simulink model "node23_case_10kV_withLoad_v2"  (R2022b)
settings: Solver=VariableStepAuto  StartTime=0.0  StopTime=10  FixedStep=1e-6  RelTol=1e-5
InitFcn:
  | sw=5;
  | Lf=1.75e-3+3.5e-3;
  | %Lf=3.5e-3;
  | %Cf=2e-4;
  | f=10;
  | Cf=15e-6;
  | % L=1.75e-3/2;
  | % X=100*pi*L;
  | % R=2*X;
  | R=0.25;X=R/0.66;
  | L=X/100/pi;
  | Z=sqrt(R^2+X^2);
  | f = 30;
  | kp1=10;
  | ki1=100;
  | kp4=20;
  | ki4=100;
  | kp16=20;
  | ki16=100;
  | % 负载参数
  | R1L=0;
  | X1L=0;
  | R2L=652.4467;
  | X2L=276.0351;
  | R3L=804.5741;
  | X3L=256.7790;
  | R4L=760.9867;
  | X4L=234.6376;
  | R5L=818.7384;
  | X5L=266.9799;
  | R6L=671.1329;
  | X6L=170.1801;
  | R7L=883.7621;
  | X7L=178.8663;
  | R8L=388.3725;
  | X8L=158.3040;
  | R9L=817.4819;
  | X9L=268.6933;
  | R10L=849.4733;
  | X10L=254.8420;
  | R11L=407.8415;
  | X11L=165.8504;
  | R12L=NaN;  % Bus 12 无 R、X 数据，用 NaN 标记
  | X12L=NaN;
  | R13L=751.2339;
  | X13L=329.8428;
  | R14L=294.0393;
  | X14L=141.6929;
  | R15L=761.9027;
  | X15L=284.3908;
  | R16L=740.4040;
  | X16L=318.2438;
  | R17L=674.5784;
  | X17L=316.4689;
  | R18L=776.7449;
  | X18L=316.6080;
  | R19L=766.0423;
  | X19L=335.7994;
  | R20L=746.0545;
  | X20L=344.3329;
  | ... (+266 lines)
libraries: spsSeriesRLCBranchLib x210, slpidlib x45, spsControlledVoltageSourceLib x30, spsThreePhaseVIMeasurementLib x24, spsPower3phInstantaneousLib x13, spsAlphaBetaZerotoabcLib x9, spsCurrentMeasurementLib x6, spsGroundLib x2, spspowerguiLib x1
(part 2 of 8)

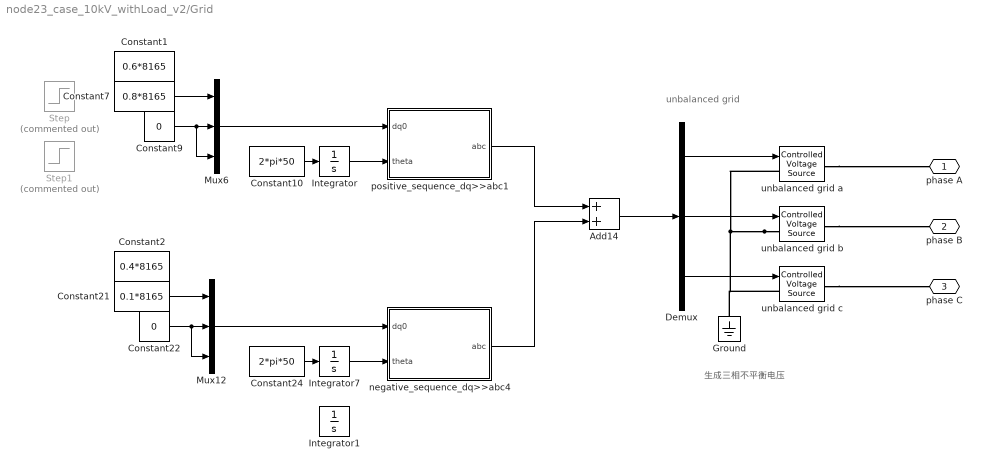
== system node23_case_10kV_withLoad_v2/Grid ==
  note: unbalanced grid
  note: 生成三相不平衡电压
  Add14 : Sum
  Constant1 : Constant  Value=0.6*8165
  Constant10 : Constant  Value=2*pi*50
  Constant2 : Constant  Value=0.4*8165
  Constant21 : Constant  Value=0.1*8165
  Constant22 : Constant  Value=0
  Constant24 : Constant  Value=2*pi*50
  Constant7 : Constant  Value=0.8*8165
  Constant9 : Constant  Value=0
  Demux : Demux  Outputs=3
  Ground : spsGroundLib/Ground  LConnTagsString=a
  Integrator : Integrator
  Integrator1 : Integrator  InitialCondition=-pi/6
  Integrator7 : Integrator  InitialCondition=-pi/2
  Mux12 : Mux  Inputs=3
  Mux6 : Mux  Inputs=3
  Step : Step  Commented=on  Time=0.25  Before=311  After=280  SampleTime=0
  Step1 : Step  Commented=on  Time=0.25  After=100  SampleTime=0
  negative_sequence_dq>>abc4 : Subsystem
  positive_sequence_dq>>abc1 : Subsystem
  unbalanced grid a : spsControlledVoltageSourceLib/Controlled Voltage Source  Initialize=on  Source_Type=AC  Amplitude=0  Phase=0  Frequency=0  Measurements=None
  "unbalanced grid b " : spsControlledVoltageSourceLib/Controlled Voltage Source  Initialize=on  Source_Type=AC  Amplitude=0  Phase=0  Frequency=0  Measurements=None
  unbalanced grid c : spsControlledVoltageSourceLib/Controlled Voltage Source  Initialize=on  Source_Type=AC  Amplitude=0  Phase=0  Frequency=0  Measurements=None
  phase A : PMIOPort  Side=Right
  phase B : PMIOPort  Port=2  Side=Right
  phase C : PMIOPort  Port=3  Side=Right
  wires:
  negative_sequence_dq>>abc4/1(abc) -> Add14/2
  Mux12/1 -> negative_sequence_dq>>abc4/1(dq0)
  Integrator/1 -> positive_sequence_dq>>abc1/2(theta)
  Demux/2 -> "unbalanced grid b "/1
  Constant24/1 -> Integrator7/1
  positive_sequence_dq>>abc1/1(abc) -> Add14/1
  Constant9/1 -> Mux6/3, Mux6/2
  Mux6/1 -> positive_sequence_dq>>abc1/1(dq0)
  Constant10/1 -> Integrator/1
  Demux/3 -> unbalanced grid c/1
  Demux/1 -> unbalanced grid a/1
  Integrator7/1 -> negative_sequence_dq>>abc4/2(theta)
  Add14/1 -> Demux/1
  Constant22/1 -> Mux12/3, Mux12/2
  Constant7/1 -> Mux6/1
  Constant21/1 -> Mux12/1
  connections:
  unbalanced grid c/RConn1 -- phase C/RConn1
  "unbalanced grid b "/LConn1 -- Ground/LConn1 -- unbalanced grid c/LConn1 -- unbalanced grid a/LConn1
  "unbalanced grid b "/RConn1 -- phase B/RConn1
  unbalanced grid a/RConn1 -- phase A/RConn1

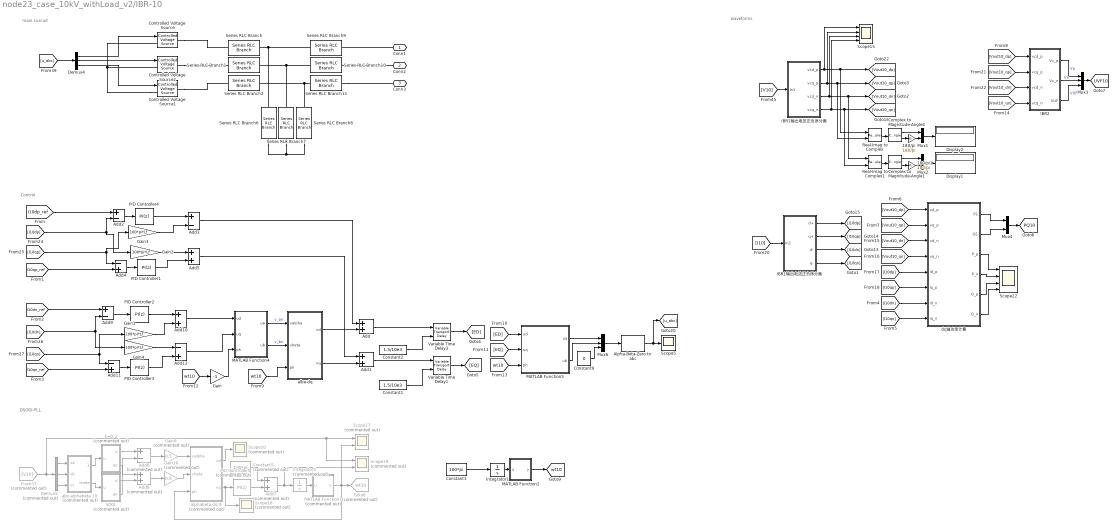
== system node23_case_10kV_withLoad_v2/IBR-10 ==
  note: DSOGI-PLL
  note: main curcuit
  note: Control
  note: waveforms
  180/pi : Gain  Gain=180/pi
  180/pi1 : Gain  Gain=180/pi
  Add{,1,5,10} (4 alike) : Sum
  Add11 : Sum  Inputs=-+
  Add12 : Sum  Inputs=-+
  Add2 : Sum  Inputs=+-
  Add3 : Sum  Inputs=+-
  Add4 : Sum  Inputs=-+
  Add6 : Sum  Commented=on  Inputs=+-
  Add7 : Sum  Commented=on
  Add8 : Sum  Commented=on
  Add9 : Sum  Inputs=+-
  Alpha-Beta-Zero to abc : spsAlphaBetaZerotoabcLib/Alpha-Beta-Zero to abc
      settings: LibrarySourceBlock=|
      | sps_lib/Control/Alpha-Beta-Zero
      | to abc
  Complex to Magnitude-Angle1 : ComplexToMagnitudeAngle
  Complex to Magnitude-Angle4 : ComplexToMagnitudeAngle
  Constant1 : Constant  Value=1.5/10e3
  Constant2 : Constant  Value=1.5/10e3
  Constant3 : Constant  Value=100*pi
  Constant5 : Constant  Commented=on  Value=100*pi
  Constant9 : Constant  Value=0
  Controlled Voltage Source : spsControlledVoltageSourceLib/Controlled Voltage Source  Initialize=on  Source_Type=AC  Amplitude=0  Phase=0  Frequency=0  Measurements=None
  Controlled Voltage Source1 : spsControlledVoltageSourceLib/Controlled Voltage Source  Initialize=on  Source_Type=AC  Amplitude=0  Phase=0  Frequency=0  Measurements=None
  Controlled Voltage Source2 : spsControlledVoltageSourceLib/Controlled Voltage Source  Initialize=on  Source_Type=AC  Amplitude=0  Phase=0  Frequency=0  Measurements=None
  Demux4 : Demux  Outputs=3
  Demux5 : Demux  Commented=on  Outputs=3
  Display1 : Display
  Display2 : Display
  From37 : From  Commented=on  GotoTag=V10  TagVisibility=global
  Gain : Gain  Gain=-1
  Gain{1..4} (4 alike) : Gain  Gain=100*pi*Lf
  Gain10 : Gain  Commented=on  Gain=0.5
  Gain9 : Gain  Commented=on  Gain=0.5
  Goto8 : Goto  Commented=on  GotoTag=wt10  TagVisibility=global
  IBR1输出电压正负序分离 : Subsystem
  IBR1输出电流正负序分离 : Subsystem
  IBR2 : MATLAB Function  TreatAsAtomicUnit=on
  Integrator1 : Integrator
  Integrator5 : Integrator  Commented=on
  MATLAB Function1 : MATLAB Function  Commented=on  TreatAsAtomicUnit=on
  MATLAB Function2 : MATLAB Function  TreatAsAtomicUnit=on
  MATLAB Function4 : MATLAB Function  TreatAsAtomicUnit=on
  MATLAB Function5 : MATLAB Function  TreatAsAtomicUnit=on
  Mux1 : Mux  Inputs=2
  Mux2 : Mux  Inputs=2
  Mux3 : Mux  Inputs=3
  Mux4 : Mux  Inputs=2
  Mux6 : Mux  Inputs=3
  PID Controller{1..4} (4 alike) : slpidlib/PID Controller  Controller=PI  Form=Parallel  TimeDomain=Discrete-time  UseExternalTs=off  SampleTime=-1  IntegratorMethod=Forward Euler  FilterMethod=Forward Euler  ControllerParametersSource=internal  P=kp1  I=ki1  UseKiTs=off  D=0  N=100  UseFilter=on  TunerSelectOption=Transfer Function Based (PID Tuner App)  InitialConditionSource=internal  InitialConditionForIntegrator=0  InitialConditionForFilter=0  DifferentiatorICPrevScaledInput=0  ExternalReset=none  TrackingMode=off  Kt=1  LimitOutput=off  SatLimitsSource=internal  UpperSaturationLimit=5  LowerSaturationLimit=-5  LinearizeAsGain=on  AntiWindupMode=none  Kb=1  LimitIntegrator=off  UpperIntegratorSaturationLimit=inf  LowerIntegratorSaturationLimit=-inf  POutMin=[]  POutMax=[]  IOutMin=[]  IOutMax=[]  DOutMin=[]  DOutMax=[]  NOutMin=[]  NOutMax=[]  SumOutMin=[]  SumOutMax=[]  SaturationOutMin=[]  SaturationOutMax=[]  PParamMin=[]  PParamMax=[]  IParamMin=[]  IParamMax=[]  DParamMin=[]  DParamMax=[]  NParamMin=[]  NParamMax=[]  KbParamMin=[]  KbParamMax=[]  KtParamMin=[]  KtParamMax=[]  KbOutMin=[]  KbOutMax=[]  KtOutMin=[]  KtOutMax=[]  IntegratorOutMin=[]  IntegratorOutMax=[]  FilterOutMin=[]  FilterOutMax=[]  SumI1OutMin=[]  SumI1OutMax=[]  SumI2OutMin=[]  SumI2OutMax=[]  SumI3OutMin=[]  SumI3OutMax=[]  SumI4OutMin=[]  SumI4OutMax=[]  SumDOutMin=[]  SumDOutMax=[]  DifferentiatorOutMin=[]  DifferentiatorOutMax=[]  FilterDiffOutCoefMin=[]  FilterDiffOutCoefMax=[]  ReciprocalOutMin=[]  ReciprocalOutMax=[]  SumDenOutMin=[]  SumDenOutMax=[]  SumNumOutMin=[]  SumNumOutMax=[]  DivideOutMin=[]  DivideOutMax=[]  UdiffTsProdOutMin=[]  UdiffTsProdOutMax=[]  NTsProdOutMin=[]  NTsProdOutMax=[]  UintegralTsProdOutMin=[]  UintegralTsProdOutMax=[]  UngainTsProdOutMin=[]  UngainTsProdOutMax=[]  ClampingZeroOutDataTypeStr=Inherit: Inherit via back propagation  ClampingZeroOutMin=[]  ClampingZeroOutMax=[]  FilterDenConstantOutDataTypeStr=Inherit: Inherit via back propagation  FilterDenConstantOutMin=[]  FilterDenConstantOutMax=[]  PCopyOutDataTypeStr=Inherit: Inherit via back propagation  PCopyOutMin=[]  PCopyOutMax=[]  NCopyOutDataTypeStr=Inherit: Inherit via back propagation  NCopyOutMin=[]  NCopyOutMax=[]  IntegratorContinuousStateAttributes=''  IntegratorStateMustResolveToSignalObject=off  IntegratorRTWStateStorageClass=Auto  FilterContinuousStateAttributes=''  FilterStateMustResolveToSignalObject=off  FilterRTWStateStorageClass=Auto  ParallelPVariant=InternalParameters  IdealPVariant=Disabled  IVariant=InternalParameters  DVariant=Disabled  IntegratorVariant=Discrete  SatVariant=Disabled  AWVariant=Passthrough  PCopyVariant=Disabled  TRVariant=Disabled  FdbkBlocksVariant=Forward  IdealPFdbkVariant=Disabled  SatFdbkVariant=Disabled  DerivativeFilterVariant=Disabled  NVariant=Disabled  NCopyVariant=Disabled_SignalSpec  FilterICVariant=Disabled  IntegratorICVariant=InternalICs  ExternalResetVariant=Disabled  TRSumVariant=Passthrough  SumFdbkVariant=Disabled  SumVariant=Sum_PI  TsampFilterVariant=InternalTs  TsampNgainVariant=Passthrough  TsampIntegralVariant=Passthrough  ExternalSaturationOutDataTypeStr=Inherit: Same as second input
  PID Controller5 : slpidlib/PID Controller  Commented=on  Controller=PI  Form=Parallel  TimeDomain=Discrete-time  UseExternalTs=off  SampleTime=-1  IntegratorMethod=Forward Euler  FilterMethod=Forward Euler  ControllerParametersSource=internal  P=1  I=3  UseKiTs=off  D=0  N=100  UseFilter=on  TunerSelectOption=Transfer Function Based (PID Tuner App)  InitialConditionSource=internal  InitialConditionForIntegrator=0  InitialConditionForFilter=0  DifferentiatorICPrevScaledInput=0  ExternalReset=none  TrackingMode=off  Kt=1  LimitOutput=off  SatLimitsSource=internal  UpperSaturationLimit=inf  LowerSaturationLimit=-inf  LinearizeAsGain=on  AntiWindupMode=none  Kb=1  LimitIntegrator=off  UpperIntegratorSaturationLimit=inf  LowerIntegratorSaturationLimit=-inf  POutMin=[]  POutMax=[]  IOutMin=[]  IOutMax=[]  DOutMin=[]  DOutMax=[]  NOutMin=[]  NOutMax=[]  SumOutMin=[]  SumOutMax=[]  SaturationOutMin=[]  SaturationOutMax=[]  PParamMin=[]  PParamMax=[]  IParamMin=[]  IParamMax=[]  DParamMin=[]  DParamMax=[]  NParamMin=[]  NParamMax=[]  KbParamMin=[]  KbParamMax=[]  KtParamMin=[]  KtParamMax=[]  KbOutMin=[]  KbOutMax=[]  KtOutMin=[]  KtOutMax=[]  IntegratorOutMin=[]  IntegratorOutMax=[]  FilterOutMin=[]  FilterOutMax=[]  SumI1OutMin=[]  SumI1OutMax=[]  SumI2OutMin=[]  SumI2OutMax=[]  SumI3OutMin=[]  SumI3OutMax=[]  SumI4OutMin=[]  SumI4OutMax=[]  SumDOutMin=[]  SumDOutMax=[]  DifferentiatorOutMin=[]  DifferentiatorOutMax=[]  FilterDiffOutCoefMin=[]  FilterDiffOutCoefMax=[]  ReciprocalOutMin=[]  ReciprocalOutMax=[]  SumDenOutMin=[]  SumDenOutMax=[]  SumNumOutMin=[]  SumNumOutMax=[]  DivideOutMin=[]  DivideOutMax=[]  UdiffTsProdOutMin=[]  UdiffTsProdOutMax=[]  NTsProdOutMin=[]  NTsProdOutMax=[]  UintegralTsProdOutMin=[]  UintegralTsProdOutMax=[]  UngainTsProdOutMin=[]  UngainTsProdOutMax=[]  ClampingZeroOutDataTypeStr=Inherit: Inherit via back propagation  ClampingZeroOutMin=[]  ClampingZeroOutMax=[]  FilterDenConstantOutDataTypeStr=Inherit: Inherit via back propagation  FilterDenConstantOutMin=[]  FilterDenConstantOutMax=[]  PCopyOutDataTypeStr=Inherit: Inherit via back propagation  PCopyOutMin=[]  PCopyOutMax=[]  NCopyOutDataTypeStr=Inherit: Inherit via back propagation  NCopyOutMin=[]  NCopyOutMax=[]  IntegratorContinuousStateAttributes=''  IntegratorStateMustResolveToSignalObject=off  IntegratorRTWStateStorageClass=Auto  FilterContinuousStateAttributes=''  FilterStateMustResolveToSignalObject=off  FilterRTWStateStorageClass=Auto  ParallelPVariant=InternalParameters  IdealPVariant=Disabled  IVariant=InternalParameters  DVariant=Disabled  IntegratorVariant=Discrete  SatVariant=Disabled  AWVariant=Passthrough  PCopyVariant=Disabled  TRVariant=Disabled  FdbkBlocksVariant=Forward  IdealPFdbkVariant=Disabled  SatFdbkVariant=Disabled  DerivativeFilterVariant=Disabled  NVariant=Disabled  NCopyVariant=Disabled_SignalSpec  FilterICVariant=Disabled  IntegratorICVariant=InternalICs  ExternalResetVariant=Disabled  TRSumVariant=Passthrough  SumFdbkVariant=Disabled  SumVariant=Sum_PI  TsampFilterVariant=InternalTs  TsampNgainVariant=Passthrough  TsampIntegralVariant=Passthrough  ExternalSaturationOutDataTypeStr=Inherit: Same as second input
  Real-Imag to Complex : RealImagToComplex
  Real-Imag to Complex1 : RealImagToComplex
  SOGI : Subsystem  Commented=on
  Scope15 : Scope  NumInputPorts=4
  Scope17 : Scope  Commented=on  NumInputPorts=2
  Scope18 : Scope  Commented=on
  Scope19 : Scope  Commented=on  NumInputPorts=2
  Scope20 : Scope  Commented=on
  Scope22 : Scope  NumInputPorts=4
  Scope5 : Scope
  Series RLC Branch : spsSeriesRLCBranchLib/Series RLC Branch  LConnTagsString=__new0  RConnTagsString=__new0  BranchType=L  Resistance=1  Inductance=3.5e-3  SetiL0=off  InitialCurrent=0  Capacitance=1e-6  Setx0=off  InitialVoltage=0  Measurements=None
  Series RLC Branch1 : spsSeriesRLCBranchLib/Series RLC Branch  LConnTagsString=__new0  RConnTagsString=__new0  BranchType=L  Resistance=1  Inductance=3.5e-3  SetiL0=off  InitialCurrent=0  Capacitance=1e-6  Setx0=off  InitialVoltage=0  Measurements=None
  Series RLC Branch10 : spsSeriesRLCBranchLib/Series RLC Branch  LConnTagsString=__new0  RConnTagsString=__new0  BranchType=L  Resistance=1  Inductance=1.75e-3  SetiL0=off  InitialCurrent=0  Capacitance=1e-6  Setx0=off  InitialVoltage=0  Measurements=None
  Series RLC Branch11 : spsSeriesRLCBranchLib/Series RLC Branch  LConnTagsString=__new0  RConnTagsString=__new0  BranchType=L  Resistance=1  Inductance=1.75e-3  SetiL0=off  InitialCurrent=0  Capacitance=1e-6  Setx0=off  InitialVoltage=0  Measurements=None
  Series RLC Branch2 : spsSeriesRLCBranchLib/Series RLC Branch  LConnTagsString=__new0  RConnTagsString=__new0  BranchType=L  Resistance=1  Inductance=3.5e-3  SetiL0=off  InitialCurrent=0  Capacitance=1e-6  Setx0=off  InitialVoltage=0  Measurements=None
  Series RLC Branch6 : spsSeriesRLCBranchLib/Series RLC Branch  LConnTagsString=__new0  RConnTagsString=__new0  BranchType=RC  Resistance=5  Inductance=500e-6  SetiL0=off  InitialCurrent=0  Capacitance=Cf  Setx0=off  InitialVoltage=0  Measurements=None
  Series RLC Branch7 : spsSeriesRLCBranchLib/Series RLC Branch  LConnTagsString=__new0  RConnTagsString=__new0  BranchType=RC  Resistance=5  Inductance=500e-6  SetiL0=off  InitialCurrent=0  Capacitance=Cf  Setx0=off  InitialVoltage=0  Measurements=None
  Series RLC Branch8 : spsSeriesRLCBranchLib/Series RLC Branch  LConnTagsString=__new0  RConnTagsString=__new0  BranchType=RC  Resistance=5  Inductance=500e-6  SetiL0=off  InitialCurrent=0  Capacitance=Cf  Setx0=off  InitialVoltage=0  Measurements=None
  Series RLC Branch9 : spsSeriesRLCBranchLib/Series RLC Branch  LConnTagsString=__new0  RConnTagsString=__new0  BranchType=L  Resistance=1  Inductance=1.75e-3  SetiL0=off  InitialCurrent=0  Capacitance=1e-6  Setx0=off  InitialVoltage=0  Measurements=None
  Variable Time Delay1 : VariableTransportDelay  MaximumDelay=10  PadeOrder=2
  Variable Time Delay3 : VariableTransportDelay  MaximumDelay=10  PadeOrder=2
  abc-alphabeta 10 : MATLAB Function  Commented=on  TreatAsAtomicUnit=on
  albe-dq : MATLAB Function  TreatAsAtomicUnit=on
  alphabeta-dq 9 : MATLAB Function  Commented=on  TreatAsAtomicUnit=on
  dq轴功率计算 : MATLAB Function  TreatAsAtomicUnit=on
  k=0.3 : Subsystem  Commented=on
  Conn1 : PMIOPort  Side=Right
  Conn2 : PMIOPort  Port=2  Side=Right
  Conn3 : PMIOPort  Port=3  Side=Right
  tag scope: PQ10=global, UVF10=global, wt10=global
  wires:
  Constant5/1 -> Add7/1
  Gain9/1 -> alphabeta-dq 9/1(valpha)
  Integrator5/1 -> MATLAB Function1/1(u)
  Add8/1 -> Gain10/1
  alphabeta-dq 9/1(vd) -> Scope20/1
  MATLAB Function1/1(y) -> alphabeta-dq 9/3(ph), Scope17/2, Goto8/1
  Add7/1 -> Scope19/2, Integrator5/1
  SOGI/1(u') -> Add8/2
  Gain10/1 -> alphabeta-dq 9/2(vbeta)
  Demux5/2 -> abc-alphabeta 10/2(vb)
  alphabeta-dq 9/2(vq) -> PID Controller5/1, Scope18/1
  Add6/1 -> Gain9/1
  From37/1 -> Demux5/1, Scope17/1, Scope19/1
  abc-alphabeta 10/1(valpha) -> k=0.3/1(u)
  abc-alphabeta 10/2(vbeta) -> SOGI/1(u)
  k=0.3/1(u') -> Add6/1
  k=0.3/2(qu') -> Add8/1
  PID Controller5/1 -> Add7/2
  Demux5/3 -> abc-alphabeta 10/3(vc)
  Demux5/1 -> abc-alphabeta 10/1(va)
  SOGI/2(qu') -> Add6/2
  Variable Time Delay3/1 -> [ED]
  Constant2/1 -> Variable Time Delay3/2
  Add1/1 -> Variable Time Delay1/1
  Add/1 -> Variable Time Delay3/1
  Constant1/1 -> Variable Time Delay1/2
  Variable Time Delay1/1 -> [EQ]
  Mux3/1 -> [UVF10]
  IBR2/3(VUF) -> Mux3/3  "VUF"
  [Vout10_dn] -> dq轴功率计算/3(vd_n)
  Complex to Magnitude-Angle4/1 -> Mux1/1
  dq轴功率计算/4(P_n) -> Scope22/2
  Mux1/1 -> Display2/1
  dq轴功率计算/6(Q_n) -> Scope22/4
  IBR1输出电压正负序分离/2(vcq_p) -> Scope15/2, [Vout10_qp], Real-Imag to Complex/2
  IBR1输出电压正负序分离/3(vcd_n) -> Scope15/3, [Vout10_dn], Real-Imag to Complex1/1
  [Vout10_qn] -> dq轴功率计算/4(vq_n)
  IBR2/2(Vc_n) -> Mux3/2  "Vn"
  Complex to Magnitude-Angle1/1 -> Mux2/1
  Mux2/1 -> Display1/1
  Mux4/1 -> [PQ10]
  Complex to Magnitude-Angle1/2 -> 180/pi1/1
  IBR1输出电压正负序分离/1(vcd_p) -> Scope15/1, Real-Imag to Complex/1, [Vout10_dp]
  180/pi1/1 -> Mux2/2
  [Vout10_qn] -> IBR2/4(vcq_n)
  [V10] -> IBR1输出电压正负序分离/1(In1)
  Real-Imag to Complex/1 -> Complex to Magnitude-Angle4/1
  180/pi/1 -> Mux1/2
  IBR1输出电流正负序分离/2(q+) -> [I10qp]
  [Vout10_dn] -> IBR2/3(vcd_n)
  [Vout10_qp] -> IBR2/2(vcq_p)
  IBR1输出电流正负序分离/4(q-) -> [I10qn]
  [Vout10_dp] -> IBR2/1(vcd_p)
  dq轴功率计算/2(Q1) -> Mux4/2
  [I10qp] -> dq轴功率计算/6(iq_p)
  [I10dn] -> dq轴功率计算/7(id_n)
  dq轴功率计算/5(Q_p) -> Scope22/3
  [I10] -> IBR1输出电流正负序分离/1(In1)
  [I10dp] -> dq轴功率计算/5(id_p)
  [Vout10_qp] -> dq轴功率计算/2(vq_p)
  [Vout10_dp] -> dq轴功率计算/1(vd_p)
  [I10qn] -> dq轴功率计算/8(iq_n)
  Real-Imag to Complex1/1 -> Complex to Magnitude-Angle1/1
  dq轴功率计算/1(P1) -> Mux4/1
  dq轴功率计算/3(P_p) -> Scope22/1
  IBR1输出电流正负序分离/3(d-) -> [I10dn]
  IBR1输出电流正负序分离/1(d+) -> [I10dp]
  IBR2/1(Vc_p) -> Mux3/1  "Vp"
  IBR1输出电压正负序分离/4(vcq_n) -> [Vout10_qn], Real-Imag to Complex1/2, Scope15/4
  Complex to Magnitude-Angle4/2 -> 180/pi/1
  [I10qn_ref] -> Add11/2
  [I10dn_ref] -> Add9/1
  [I10qp_ref] -> Add4/2
  [I10dp_ref] -> Add2/1
  MATLAB Function5/1(ua) -> Mux6/1
  Constant9/1 -> Mux6/3
  Alpha-Beta-Zero to abc/1 -> Scope5/1, [u_abc]
  Mux6/1 -> Alpha-Beta-Zero to abc/1
  [u_abc] -> Demux4/1
  Demux4/1 -> Controlled Voltage Source/1
  Demux4/2 -> Controlled Voltage Source2/1
  Demux4/3 -> Controlled Voltage Source1/1
  [wt10] -> Gain/1
  MATLAB Function4/1(ua) -> albe-dq/1(valpha)  "v_an"
  [I10qn] -> Add11/1, Gain1/1
  [I10dn] -> Add9/2, Gain4/1
  PID Controller1/1 -> Add5/2
  albe-dq/2(vq) -> Add1/2
  Gain1/1 -> Add10/2
  Add5/1 -> Add1/1
  albe-dq/1(vd) -> Add/2
  Gain2/1 -> Add5/1
  [I10qp] -> Gain3/1, Add4/1
  [wt10] -> albe-dq/3(ph)
  PID Controller4/1 -> Add3/1
  Gain3/1 -> Add3/2
  Add4/1 -> PID Controller1/1
  [ED] -> MATLAB Function5/1(ud)
  Add11/1 -> PID Controller3/1
  Add10/1 -> MATLAB Function4/1(ud)
  Add2/1 -> PID Controller4/1
  MATLAB Function4/2(ub) -> albe-dq/2(vbeta)  "v_bn"
  MATLAB Function5/2(ub) -> Mux6/2
  Add9/1 -> PID Controller2/1
  Gain/1 -> MATLAB Function4/3(ph)
  Gain4/1 -> Add12/1
  [I10dp] -> Add2/2, Gain2/1
  PID Controller2/1 -> Add10/1
  PID Controller3/1 -> Add12/2
  Add3/1 -> Add/1
  [wt10] -> MATLAB Function5/3(ph)
  Add12/1 -> MATLAB Function4/2(uq)
  [EQ] -> MATLAB Function5/2(uq)
  Constant3/1 -> Integrator1/1
  MATLAB Function2/1(y) -> [wt10]
  Integrator1/1 -> MATLAB Function2/1(u)
  connections:
  Controlled Voltage Source1/LConn1 -- Controlled Voltage Source2/LConn1 -- Controlled Voltage Source/LConn1
  Conn1/RConn1 -- Series RLC Branch9/RConn1
  Series RLC Branch10/RConn1 -- Conn2/RConn1
  Series RLC Branch11/RConn1 -- Conn3/RConn1
  Controlled Voltage Source/RConn1 -- Series RLC Branch/LConn1
  Series RLC Branch8/RConn1 -- Series RLC Branch6/RConn1 -- Series RLC Branch7/RConn1
  Controlled Voltage Source1/RConn1 -- Series RLC Branch2/LConn1
  Controlled Voltage Source2/RConn1 -- Series RLC Branch1/LConn1
  Series RLC Branch/RConn1 -- Series RLC Branch6/LConn1 -- Series RLC Branch9/LConn1
  Series RLC Branch1/RConn1 -- Series RLC Branch7/LConn1 -- Series RLC Branch10/LConn1
  Series RLC Branch8/LConn1 -- Series RLC Branch2/RConn1 -- Series RLC Branch11/LConn1

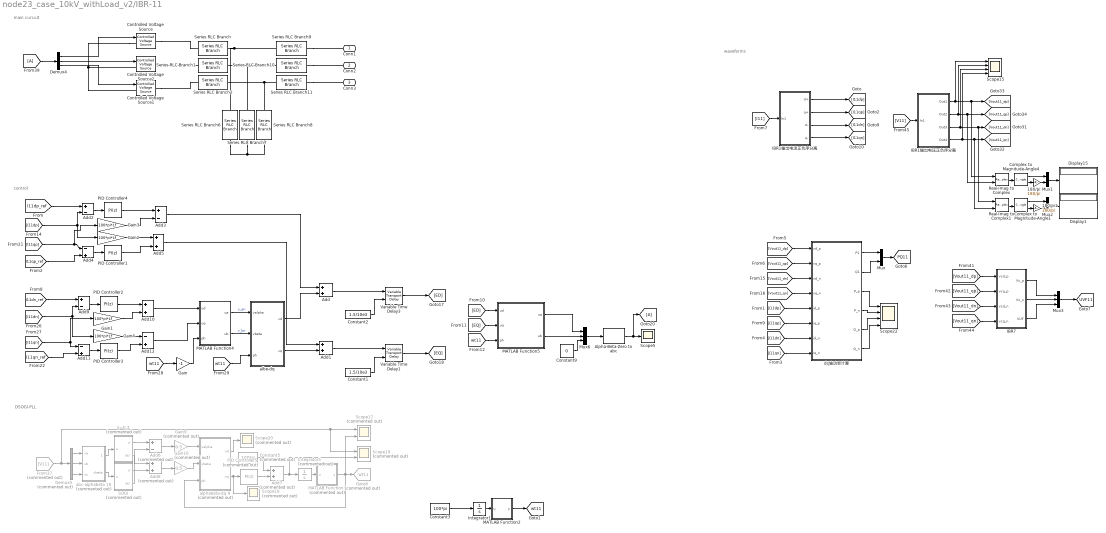
== system node23_case_10kV_withLoad_v2/IBR-11 ==
  note: waveforms
  note: DSOGI-PLL
  note: control
  note: main curcuit
  180/pi : Gain  Gain=180/pi
  180/pi1 : Gain  Gain=180/pi
  Add{,1,5,10} (4 alike) : Sum
  Add11 : Sum  Inputs=-+
  Add12 : Sum  Inputs=-+
  Add2 : Sum  Inputs=+-
  Add3 : Sum  Inputs=+-
  Add4 : Sum  Inputs=-+
  Add6 : Sum  Commented=on  Inputs=+-
  Add7 : Sum  Commented=on
  Add8 : Sum  Commented=on
  Add9 : Sum  Inputs=+-
  Alpha-Beta-Zero to abc : spsAlphaBetaZerotoabcLib/Alpha-Beta-Zero to abc
      settings: LibrarySourceBlock=|
      | sps_lib/Control/Alpha-Beta-Zero
      | to abc
  Complex to Magnitude-Angle1 : ComplexToMagnitudeAngle
  Complex to Magnitude-Angle4 : ComplexToMagnitudeAngle
  Constant1 : Constant  Value=1.5/10e3
  Constant2 : Constant  Value=1.5/10e3
  Constant3 : Constant  Value=100*pi
  Constant5 : Constant  Commented=on  Value=100*pi
  Constant9 : Constant  Value=0
  Controlled Voltage Source : spsControlledVoltageSourceLib/Controlled Voltage Source  Initialize=on  Source_Type=AC  Amplitude=0  Phase=0  Frequency=0  Measurements=None
  Controlled Voltage Source1 : spsControlledVoltageSourceLib/Controlled Voltage Source  Initialize=on  Source_Type=AC  Amplitude=0  Phase=0  Frequency=0  Measurements=None
  Controlled Voltage Source2 : spsControlledVoltageSourceLib/Controlled Voltage Source  Initialize=on  Source_Type=AC  Amplitude=0  Phase=0  Frequency=0  Measurements=None
  Demux4 : Demux  Outputs=3
  Demux5 : Demux  Commented=on  Outputs=3
  Display1 : Display
  Display15 : Display
  From37 : From  Commented=on  GotoTag=V11  TagVisibility=global
  From39 : From
  Gain : Gain  Gain=-1
  Gain{1..4} (4 alike) : Gain  Gain=100*pi*Lf
  Gain10 : Gain  Commented=on  Gain=0.5
  Gain9 : Gain  Commented=on  Gain=0.5
  Goto20 : Goto
  Goto8 : Goto  Commented=on  GotoTag=wt11  TagVisibility=global
  IBR1输出电压正负序分离 : Subsystem
  IBR1输出电流正负序分离 : Subsystem
  IBR7 : MATLAB Function  TreatAsAtomicUnit=on
  Integrator1 : Integrator
  Integrator5 : Integrator  Commented=on
  MATLAB Function1 : MATLAB Function  Commented=on  TreatAsAtomicUnit=on
  MATLAB Function2 : MATLAB Function  TreatAsAtomicUnit=on
  MATLAB Function4 : MATLAB Function  TreatAsAtomicUnit=on
  MATLAB Function5 : MATLAB Function  TreatAsAtomicUnit=on
  Mux : Mux  Inputs=2
  Mux1 : Mux  Inputs=2
  Mux2 : Mux  Inputs=2
  Mux3 : Mux  Inputs=3
  Mux6 : Mux  Inputs=3
  PID Controller{1..4} (4 alike) : slpidlib/PID Controller  Controller=PI  Form=Parallel  TimeDomain=Discrete-time  UseExternalTs=off  SampleTime=-1  IntegratorMethod=Forward Euler  FilterMethod=Forward Euler  ControllerParametersSource=internal  P=kp1  I=ki1  UseKiTs=off  D=0  N=100  UseFilter=on  TunerSelectOption=Transfer Function Based (PID Tuner App)  InitialConditionSource=internal  InitialConditionForIntegrator=0  InitialConditionForFilter=0  DifferentiatorICPrevScaledInput=0  ExternalReset=none  TrackingMode=off  Kt=1  LimitOutput=off  SatLimitsSource=internal  UpperSaturationLimit=5  LowerSaturationLimit=-5  LinearizeAsGain=on  AntiWindupMode=none  Kb=1  LimitIntegrator=off  UpperIntegratorSaturationLimit=inf  LowerIntegratorSaturationLimit=-inf  POutMin=[]  POutMax=[]  IOutMin=[]  IOutMax=[]  DOutMin=[]  DOutMax=[]  NOutMin=[]  NOutMax=[]  SumOutMin=[]  SumOutMax=[]  SaturationOutMin=[]  SaturationOutMax=[]  PParamMin=[]  PParamMax=[]  IParamMin=[]  IParamMax=[]  DParamMin=[]  DParamMax=[]  NParamMin=[]  NParamMax=[]  KbParamMin=[]  KbParamMax=[]  KtParamMin=[]  KtParamMax=[]  KbOutMin=[]  KbOutMax=[]  KtOutMin=[]  KtOutMax=[]  IntegratorOutMin=[]  IntegratorOutMax=[]  FilterOutMin=[]  FilterOutMax=[]  SumI1OutMin=[]  SumI1OutMax=[]  SumI2OutMin=[]  SumI2OutMax=[]  SumI3OutMin=[]  SumI3OutMax=[]  SumI4OutMin=[]  SumI4OutMax=[]  SumDOutMin=[]  SumDOutMax=[]  DifferentiatorOutMin=[]  DifferentiatorOutMax=[]  FilterDiffOutCoefMin=[]  FilterDiffOutCoefMax=[]  ReciprocalOutMin=[]  ReciprocalOutMax=[]  SumDenOutMin=[]  SumDenOutMax=[]  SumNumOutMin=[]  SumNumOutMax=[]  DivideOutMin=[]  DivideOutMax=[]  UdiffTsProdOutMin=[]  UdiffTsProdOutMax=[]  NTsProdOutMin=[]  NTsProdOutMax=[]  UintegralTsProdOutMin=[]  UintegralTsProdOutMax=[]  UngainTsProdOutMin=[]  UngainTsProdOutMax=[]  ClampingZeroOutDataTypeStr=Inherit: Inherit via back propagation  ClampingZeroOutMin=[]  ClampingZeroOutMax=[]  FilterDenConstantOutDataTypeStr=Inherit: Inherit via back propagation  FilterDenConstantOutMin=[]  FilterDenConstantOutMax=[]  PCopyOutDataTypeStr=Inherit: Inherit via back propagation  PCopyOutMin=[]  PCopyOutMax=[]  NCopyOutDataTypeStr=Inherit: Inherit via back propagation  NCopyOutMin=[]  NCopyOutMax=[]  IntegratorContinuousStateAttributes=''  IntegratorStateMustResolveToSignalObject=off  IntegratorRTWStateStorageClass=Auto  FilterContinuousStateAttributes=''  FilterStateMustResolveToSignalObject=off  FilterRTWStateStorageClass=Auto  ParallelPVariant=InternalParameters  IdealPVariant=Disabled  IVariant=InternalParameters  DVariant=Disabled  IntegratorVariant=Discrete  SatVariant=Disabled  AWVariant=Passthrough  PCopyVariant=Disabled  TRVariant=Disabled  FdbkBlocksVariant=Forward  IdealPFdbkVariant=Disabled  SatFdbkVariant=Disabled  DerivativeFilterVariant=Disabled  NVariant=Disabled  NCopyVariant=Disabled_SignalSpec  FilterICVariant=Disabled  IntegratorICVariant=InternalICs  ExternalResetVariant=Disabled  TRSumVariant=Passthrough  SumFdbkVariant=Disabled  SumVariant=Sum_PI  TsampFilterVariant=InternalTs  TsampNgainVariant=Passthrough  TsampIntegralVariant=Passthrough  ExternalSaturationOutDataTypeStr=Inherit: Same as second input
  PID Controller5 : slpidlib/PID Controller  Commented=on  Controller=PI  Form=Parallel  TimeDomain=Discrete-time  UseExternalTs=off  SampleTime=-1  IntegratorMethod=Forward Euler  FilterMethod=Forward Euler  ControllerParametersSource=internal  P=1  I=3  UseKiTs=off  D=0  N=100  UseFilter=on  TunerSelectOption=Transfer Function Based (PID Tuner App)  InitialConditionSource=internal  InitialConditionForIntegrator=0  InitialConditionForFilter=0  DifferentiatorICPrevScaledInput=0  ExternalReset=none  TrackingMode=off  Kt=1  LimitOutput=off  SatLimitsSource=internal  UpperSaturationLimit=inf  LowerSaturationLimit=-inf  LinearizeAsGain=on  AntiWindupMode=none  Kb=1  LimitIntegrator=off  UpperIntegratorSaturationLimit=inf  LowerIntegratorSaturationLimit=-inf  POutMin=[]  POutMax=[]  IOutMin=[]  IOutMax=[]  DOutMin=[]  DOutMax=[]  NOutMin=[]  NOutMax=[]  SumOutMin=[]  SumOutMax=[]  SaturationOutMin=[]  SaturationOutMax=[]  PParamMin=[]  PParamMax=[]  IParamMin=[]  IParamMax=[]  DParamMin=[]  DParamMax=[]  NParamMin=[]  NParamMax=[]  KbParamMin=[]  KbParamMax=[]  KtParamMin=[]  KtParamMax=[]  KbOutMin=[]  KbOutMax=[]  KtOutMin=[]  KtOutMax=[]  IntegratorOutMin=[]  IntegratorOutMax=[]  FilterOutMin=[]  FilterOutMax=[]  SumI1OutMin=[]  SumI1OutMax=[]  SumI2OutMin=[]  SumI2OutMax=[]  SumI3OutMin=[]  SumI3OutMax=[]  SumI4OutMin=[]  SumI4OutMax=[]  SumDOutMin=[]  SumDOutMax=[]  DifferentiatorOutMin=[]  DifferentiatorOutMax=[]  FilterDiffOutCoefMin=[]  FilterDiffOutCoefMax=[]  ReciprocalOutMin=[]  ReciprocalOutMax=[]  SumDenOutMin=[]  SumDenOutMax=[]  SumNumOutMin=[]  SumNumOutMax=[]  DivideOutMin=[]  DivideOutMax=[]  UdiffTsProdOutMin=[]  UdiffTsProdOutMax=[]  NTsProdOutMin=[]  NTsProdOutMax=[]  UintegralTsProdOutMin=[]  UintegralTsProdOutMax=[]  UngainTsProdOutMin=[]  UngainTsProdOutMax=[]  ClampingZeroOutDataTypeStr=Inherit: Inherit via back propagation  ClampingZeroOutMin=[]  ClampingZeroOutMax=[]  FilterDenConstantOutDataTypeStr=Inherit: Inherit via back propagation  FilterDenConstantOutMin=[]  FilterDenConstantOutMax=[]  PCopyOutDataTypeStr=Inherit: Inherit via back propagation  PCopyOutMin=[]  PCopyOutMax=[]  NCopyOutDataTypeStr=Inherit: Inherit via back propagation  NCopyOutMin=[]  NCopyOutMax=[]  IntegratorContinuousStateAttributes=''  IntegratorStateMustResolveToSignalObject=off  IntegratorRTWStateStorageClass=Auto  FilterContinuousStateAttributes=''  FilterStateMustResolveToSignalObject=off  FilterRTWStateStorageClass=Auto  ParallelPVariant=InternalParameters  IdealPVariant=Disabled  IVariant=InternalParameters  DVariant=Disabled  IntegratorVariant=Discrete  SatVariant=Disabled  AWVariant=Passthrough  PCopyVariant=Disabled  TRVariant=Disabled  FdbkBlocksVariant=Forward  IdealPFdbkVariant=Disabled  SatFdbkVariant=Disabled  DerivativeFilterVariant=Disabled  NVariant=Disabled  NCopyVariant=Disabled_SignalSpec  FilterICVariant=Disabled  IntegratorICVariant=InternalICs  ExternalResetVariant=Disabled  TRSumVariant=Passthrough  SumFdbkVariant=Disabled  SumVariant=Sum_PI  TsampFilterVariant=InternalTs  TsampNgainVariant=Passthrough  TsampIntegralVariant=Passthrough  ExternalSaturationOutDataTypeStr=Inherit: Same as second input
  Real-Imag to Complex : RealImagToComplex
  Real-Imag to Complex1 : RealImagToComplex
  SOGI : Subsystem  Commented=on
  Scope15 : Scope  NumInputPorts=4
  Scope17 : Scope  Commented=on  NumInputPorts=2
  Scope18 : Scope  Commented=on
  Scope19 : Scope  Commented=on  NumInputPorts=2
  Scope20 : Scope  Commented=on
  Scope22 : Scope  NumInputPorts=4
  Scope5 : Scope
  Series RLC Branch : spsSeriesRLCBranchLib/Series RLC Branch  LConnTagsString=__new0  RConnTagsString=__new0  BranchType=L  Resistance=1  Inductance=3.5e-3  SetiL0=off  InitialCurrent=0  Capacitance=1e-6  Setx0=off  InitialVoltage=0  Measurements=None
  Series RLC Branch1 : spsSeriesRLCBranchLib/Series RLC Branch  LConnTagsString=__new0  RConnTagsString=__new0  BranchType=L  Resistance=1  Inductance=3.5e-3  SetiL0=off  InitialCurrent=0  Capacitance=1e-6  Setx0=off  InitialVoltage=0  Measurements=None
  Series RLC Branch10 : spsSeriesRLCBranchLib/Series RLC Branch  LConnTagsString=__new0  RConnTagsString=__new0  BranchType=L  Resistance=1  Inductance=1.75e-3  SetiL0=off  InitialCurrent=0  Capacitance=1e-6  Setx0=off  InitialVoltage=0  Measurements=None
  Series RLC Branch11 : spsSeriesRLCBranchLib/Series RLC Branch  LConnTagsString=__new0  RConnTagsString=__new0  BranchType=L  Resistance=1  Inductance=1.75e-3  SetiL0=off  InitialCurrent=0  Capacitance=1e-6  Setx0=off  InitialVoltage=0  Measurements=None
  Series RLC Branch2 : spsSeriesRLCBranchLib/Series RLC Branch  LConnTagsString=__new0  RConnTagsString=__new0  BranchType=L  Resistance=1  Inductance=3.5e-3  SetiL0=off  InitialCurrent=0  Capacitance=1e-6  Setx0=off  InitialVoltage=0  Measurements=None
  Series RLC Branch6 : spsSeriesRLCBranchLib/Series RLC Branch  LConnTagsString=__new0  RConnTagsString=__new0  BranchType=RC  Resistance=5  Inductance=500e-6  SetiL0=off  InitialCurrent=0  Capacitance=Cf  Setx0=off  InitialVoltage=0  Measurements=None
  Series RLC Branch7 : spsSeriesRLCBranchLib/Series RLC Branch  LConnTagsString=__new0  RConnTagsString=__new0  BranchType=RC  Resistance=5  Inductance=500e-6  SetiL0=off  InitialCurrent=0  Capacitance=Cf  Setx0=off  InitialVoltage=0  Measurements=None
  Series RLC Branch8 : spsSeriesRLCBranchLib/Series RLC Branch  LConnTagsString=__new0  RConnTagsString=__new0  BranchType=RC  Resistance=5  Inductance=500e-6  SetiL0=off  InitialCurrent=0  Capacitance=Cf  Setx0=off  InitialVoltage=0  Measurements=None
  Series RLC Branch9 : spsSeriesRLCBranchLib/Series RLC Branch  LConnTagsString=__new0  RConnTagsString=__new0  BranchType=L  Resistance=1  Inductance=1.75e-3  SetiL0=off  InitialCurrent=0  Capacitance=1e-6  Setx0=off  InitialVoltage=0  Measurements=None
  Variable Time Delay1 : VariableTransportDelay  MaximumDelay=10  PadeOrder=2
  Variable Time Delay3 : VariableTransportDelay  MaximumDelay=10  PadeOrder=2
  abc-alphabeta 10 : MATLAB Function  Commented=on  TreatAsAtomicUnit=on
  albe-dq : MATLAB Function  TreatAsAtomicUnit=on
  alphabeta-dq 9 : MATLAB Function  Commented=on  TreatAsAtomicUnit=on
  dq轴功率计算 : MATLAB Function  TreatAsAtomicUnit=on
  k=0.3 : Subsystem  Commented=on
  Conn1 : PMIOPort  Side=Right
  Conn2 : PMIOPort  Port=2  Side=Right
  Conn3 : PMIOPort  Port=3  Side=Right
  tag scope: PQ11=global, UVF11=global, wt11=global
  wires:
  IBR1输出电压正负序分离/4(Out4) -> [Vout11_qn], Real-Imag to Complex1/2, Scope15/4
  Complex to Magnitude-Angle1/1 -> Mux2/1
  Complex to Magnitude-Angle1/2 -> 180/pi1/1
  Real-Imag to Complex1/1 -> Complex to Magnitude-Angle1/1
  180/pi1/1 -> Mux2/2
  Mux2/1 -> Display1/1
  IBR1输出电压正负序分离/1(Out1) -> Scope15/1, [Vout11_dp], Real-Imag to Complex/1
  Mux1/1 -> Display15/1
  180/pi/1 -> Mux1/2
  Real-Imag to Complex/1 -> Complex to Magnitude-Angle4/1
  Complex to Magnitude-Angle4/2 -> 180/pi/1
  Complex to Magnitude-Angle4/1 -> Mux1/1
  Mux/1 -> [PQ11]
  [I11dn] -> dq轴功率计算/7(id_n)
  [I11qp] -> dq轴功率计算/6(iq_p)
  [I11dp] -> dq轴功率计算/5(id_p)
  [Vout11_qn] -> dq轴功率计算/4(vq_n)
  [Vout11_dn] -> dq轴功率计算/3(vd_n)
  [Vout11_qp] -> dq轴功率计算/2(vq_p)
  [I11qn] -> dq轴功率计算/8(iq_n)
  [Vout11_dp] -> dq轴功率计算/1(vd_p)
  dq轴功率计算/2(Q1) -> Mux/2
  dq轴功率计算/3(P_p) -> Scope22/1
  dq轴功率计算/5(Q_p) -> Scope22/3
  dq轴功率计算/4(P_n) -> Scope22/2
  dq轴功率计算/6(Q_n) -> Scope22/4
  dq轴功率计算/1(P1) -> Mux/1
  [wt11] -> Gain/1
  MATLAB Function4/1(ua) -> albe-dq/1(valpha)  "v_an"
  [I11qn] -> Add11/1, Gain1/1
  [I11dn] -> Gain4/1, Add9/2
  PID Controller1/1 -> Add5/2
  albe-dq/2(vq) -> Add1/2
  Gain1/1 -> Add10/2
  Add5/1 -> Add1/1
  albe-dq/1(vd) -> Add/2
  Gain2/1 -> Add5/1
  [I11qp] -> Add4/1, Gain3/1
  [wt11] -> albe-dq/3(ph)
  PID Controller4/1 -> Add3/1
  Gain3/1 -> Add3/2
  Add4/1 -> PID Controller1/1
  [ED] -> MATLAB Function5/1(ud)
  Add11/1 -> PID Controller3/1
  Add10/1 -> MATLAB Function4/1(ud)
  MATLAB Function4/2(ub) -> albe-dq/2(vbeta)  "v_bn"
  MATLAB Function5/2(ub) -> Mux6/2
  Add9/1 -> PID Controller2/1
  Gain/1 -> MATLAB Function4/3(ph)
  Gain4/1 -> Add12/1
  [I11dp] -> Add2/2, Gain2/1
  PID Controller2/1 -> Add10/1
  PID Controller3/1 -> Add12/2
  Add3/1 -> Add/1
  [wt11] -> MATLAB Function5/3(ph)
  Add12/1 -> MATLAB Function4/2(uq)
  [EQ] -> MATLAB Function5/2(uq)
  [Vout11_qn] -> IBR7/4(vcq_n)
  [Vout11_dp] -> IBR7/1(vcd_p)
  [Vout11_qp] -> IBR7/2(vcq_p)
  [Vout11_dn] -> IBR7/3(vcd_n)
  [I11] -> IBR1输出电流正负序分离/1(In1)
  IBR1输出电流正负序分离/1(d+) -> [I11dp]
  IBR1输出电压正负序分离/2(Out2) -> [Vout11_qp], Real-Imag to Complex/2, Scope15/2
  [V11] -> IBR1输出电压正负序分离/1(In1)
  IBR1输出电流正负序分离/4(q-) -> [I11qn]
  IBR1输出电压正负序分离/3(Out3) -> Scope15/3, [Vout11_dn], Real-Imag to Complex1/1
  IBR7/2(Vc_n) -> Mux3/2
  IBR7/1(Vc_p) -> Mux3/1
  IBR7/3(VUF) -> Mux3/3
  Mux3/1 -> [UVF11]
  Add2/1 -> PID Controller4/1
  MATLAB Function5/1(ua) -> Mux6/1
  Mux6/1 -> Alpha-Beta-Zero to abc/1
  Alpha-Beta-Zero to abc/1 -> Goto20/1, Scope5/1
  Constant9/1 -> Mux6/3
  From39/1 -> Demux4/1
  Demux4/2 -> Controlled Voltage Source2/1
  Demux4/3 -> Controlled Voltage Source1/1
  Demux4/1 -> Controlled Voltage Source/1
  [I11qn_ref] -> Add11/2
  [I11dn_ref] -> Add9/1
  [I11qp_ref] -> Add4/2
  [I11dp_ref] -> Add2/1
  IBR1输出电流正负序分离/2(q+) -> [I11qp]
  IBR1输出电流正负序分离/3(d-) -> [I11dn]
  Add/1 -> Variable Time Delay3/1
  Constant2/1 -> Variable Time Delay3/2
  Variable Time Delay3/1 -> [ED]
  Constant1/1 -> Variable Time Delay1/2
  Add1/1 -> Variable Time Delay1/1
  Variable Time Delay1/1 -> [EQ]
  Add8/1 -> Gain10/1
  Gain9/1 -> alphabeta-dq 9/1(valpha)
  Integrator5/1 -> MATLAB Function1/1(u)
  MATLAB Function1/1(y) -> Goto8/1, Scope17/2, alphabeta-dq 9/3(ph)
  Constant5/1 -> Add7/1
  alphabeta-dq 9/1(vd) -> Scope20/1
  From37/1 -> Scope19/1, Scope17/1, Demux5/1
  Gain10/1 -> alphabeta-dq 9/2(vbeta)
  alphabeta-dq 9/2(vq) -> Scope18/1, PID Controller5/1
  SOGI/1(u') -> Add8/2
  Add7/1 -> Integrator5/1, Scope19/2
  k=0.3/1(u') -> Add6/1
  Add6/1 -> Gain9/1
  abc-alphabeta 10/1(valpha) -> k=0.3/1(u)
  Demux5/2 -> abc-alphabeta 10/2(vb)
  Demux5/1 -> abc-alphabeta 10/1(va)
  k=0.3/2(qu') -> Add8/1
  Demux5/3 -> abc-alphabeta 10/3(vc)
  SOGI/2(qu') -> Add6/2
  abc-alphabeta 10/2(vbeta) -> SOGI/1(u)
  PID Controller5/1 -> Add7/2
  Constant3/1 -> Integrator1/1
  MATLAB Function2/1(y) -> [wt11]
  Integrator1/1 -> MATLAB Function2/1(u)
  connections:
  Series RLC Branch9/RConn1 -- Conn1/RConn1
  Series RLC Branch10/RConn1 -- Conn2/RConn1
  Series RLC Branch11/RConn1 -- Conn3/RConn1
  Controlled Voltage Source/RConn1 -- Series RLC Branch/LConn1
  Series RLC Branch8/RConn1 -- Series RLC Branch7/RConn1 -- Series RLC Branch6/RConn1
  Controlled Voltage Source1/RConn1 -- Series RLC Branch2/LConn1
  Controlled Voltage Source2/RConn1 -- Series RLC Branch1/LConn1
  Series RLC Branch9/LConn1 -- Series RLC Branch6/LConn1 -- Series RLC Branch/RConn1
  Series RLC Branch10/LConn1 -- Series RLC Branch1/RConn1 -- Series RLC Branch7/LConn1
  Series RLC Branch11/LConn1 -- Series RLC Branch2/RConn1 -- Series RLC Branch8/LConn1
  Controlled Voltage Source/LConn1 -- Controlled Voltage Source2/LConn1 -- Controlled Voltage Source1/LConn1
